simulink model "StSys_StrtCtl"  (R2016b)
settings: configuration reference "CodeGenConfigSet" (kept outside this file)
values from neighbouring files (symbols this model uses):
  Strt_uThresIniMinStrt_C = Calibration.Parameter    [init_StSys_StrtCtl.m]    (also in init_StSys_StrtCtl_SIL.m = Simulink.Parameter)
  StSys_nBlnd_C = Calibration.Parameter    [init_StSys_StrtCtl.m]    (also in init_StSys_StrtCtl_SIL.m = Simulink.Parameter)
  StSys_nThres_C = Calibration.Parameter    [init_StSys_StrtCtl.m]    (also in init_StSys_StrtCtl_SIL.m = Simulink.Parameter)
  StSys_nThresCalc_CUR = Calibration.Parameter    [init_StSys_StrtCtl.m]    (also in init_StSys_StrtCtl_SIL.m = Simulink.Parameter)
  StSys_nThresCalc_CURX = Calibration.Parameter    [init_StSys_StrtCtl.m]    (also in init_StSys_StrtCtl_SIL.m = Simulink.Parameter)
  StSys_stCondActv_C = Calibration.Parameter    [init_StSys_StrtCtl.m]    (also in init_StSys_StrtCtl_SIL.m = Simulink.Parameter)
  StSys_stCondDeactv_C = Calibration.Parameter    [init_StSys_StrtCtl.m]    (also in init_StSys_StrtCtl_SIL.m = Simulink.Parameter)
  StSys_stLogicT50CAN_C = Calibration.Parameter    [init_StSys_StrtCtl.m]    (also in init_StSys_StrtCtl_SIL.m = Simulink.Parameter)
  StSys_stLogicT50EMGCY_C = Calibration.Parameter    [init_StSys_StrtCtl.m]    (also in init_StSys_StrtCtl_SIL.m = Simulink.Parameter)
  StSys_stLogicT50NRM_C = Calibration.Parameter    [init_StSys_StrtCtl.m]    (also in init_StSys_StrtCtl_SIL.m = Simulink.Parameter)
  StSys_stSelectT50CAN_C = Calibration.Parameter    [init_StSys_StrtCtl.m]    (also in init_StSys_StrtCtl_SIL.m = Simulink.Parameter)
  StSys_stSelectT50EMGCY_C = Calibration.Parameter    [init_StSys_StrtCtl.m]    (also in init_StSys_StrtCtl_SIL.m = Simulink.Parameter)
  StSys_stSelectT50NRM_C = Calibration.Parameter    [init_StSys_StrtCtl.m]    (also in init_StSys_StrtCtl_SIL.m = Simulink.Parameter)
  StSys_tiBlnd_C = Calibration.Parameter    [init_StSys_StrtCtl.m]    (also in init_StSys_StrtCtl_SIL.m = Simulink.Parameter)
  StSys_tiStrtON_C = Calibration.Parameter    [init_StSys_StrtCtl.m]    (also in init_StSys_StrtCtl_SIL.m = Simulink.Parameter)
  StSys_vEngCompStrt_C = Calibration.Parameter    [init_StSys_StrtCtl.m]    (also in init_StSys_StrtCtl_SIL.m = Simulink.Parameter)
  StSys_vThresT50CAN_C = Calibration.Parameter    [init_StSys_StrtCtl.m]    (also in init_StSys_StrtCtl_SIL.m = Simulink.Parameter)
  StSys_vThresT50EMGCY_C = Calibration.Parameter    [init_StSys_StrtCtl.m]    (also in init_StSys_StrtCtl_SIL.m = Simulink.Parameter)
  StSys_vThresT50NRM_C = Calibration.Parameter    [init_StSys_StrtCtl.m]    (also in init_StSys_StrtCtl_SIL.m = Simulink.Parameter)
undefined symbols (not defined in the file or in its folder): AirHtState_conv, StSys_StrtCtl_DT, StSys_StrtState_conv
libraries: simulink x201, CXLib x7
(part 2 of 2)

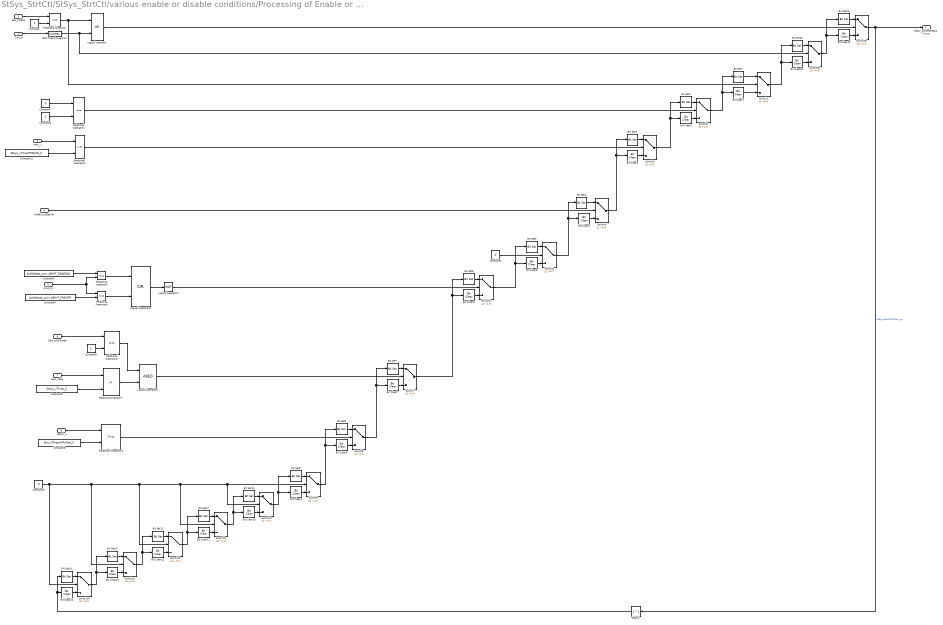
== system StSys_StrtCtl/StSys_StrtCtl/various enable or disable conditions/Processing of Enable or disable conditions for T50CAN ==
  Gbx_stNPos : Inport
  Clth_st : Inport  Port=2
  VehV_v : Inport  Port=3
  HndBrk_stDebVal : Inport  Port=4
  AirHt_st : Inport  Port=5
  Epm_stOpMode : Inport  Port=6
  Epm_nEng : Inport  Port=7
  BattU_u : Inport  Port=8
  Bit Clear1 : simulink/Logic and Bit Operations/Bit Clear  iBit=2
  Bit Clear10 : simulink/Logic and Bit Operations/Bit Clear  iBit=11
  Bit Clear11 : simulink/Logic and Bit Operations/Bit Clear  iBit=12
  Bit Clear12 : simulink/Logic and Bit Operations/Bit Clear  iBit=13
  Bit Clear13 : simulink/Logic and Bit Operations/Bit Clear  iBit=14
  Bit Clear14 : simulink/Logic and Bit Operations/Bit Clear  iBit=15
  Bit Clear2 : simulink/Logic and Bit Operations/Bit Clear  iBit=3
  Bit Clear3 : simulink/Logic and Bit Operations/Bit Clear  iBit=4
  Bit Clear4 : simulink/Logic and Bit Operations/Bit Clear  iBit=5
  Bit Clear41 : simulink/Logic and Bit Operations/Bit Clear  iBit=0
  Bit Clear5 : simulink/Logic and Bit Operations/Bit Clear  iBit=6
  Bit Clear54 : simulink/Logic and Bit Operations/Bit Clear  iBit=1
  Bit Clear6 : simulink/Logic and Bit Operations/Bit Clear  iBit=7
  Bit Clear7 : simulink/Logic and Bit Operations/Bit Clear  iBit=8
  Bit Clear8 : simulink/Logic and Bit Operations/Bit Clear  iBit=9
  Bit Clear9 : simulink/Logic and Bit Operations/Bit Clear  iBit=10
  Bit Set1 : simulink/Logic and Bit Operations/Bit Set  iBit=2
  Bit Set10 : simulink/Logic and Bit Operations/Bit Set  iBit=11
  Bit Set11 : simulink/Logic and Bit Operations/Bit Set  iBit=12
  Bit Set12 : simulink/Logic and Bit Operations/Bit Set  iBit=13
  Bit Set13 : simulink/Logic and Bit Operations/Bit Set  iBit=14
  Bit Set14 : simulink/Logic and Bit Operations/Bit Set  iBit=15
  Bit Set18 : simulink/Logic and Bit Operations/Bit Set  iBit=1
  Bit Set2 : simulink/Logic and Bit Operations/Bit Set  iBit=3
  Bit Set24 : simulink/Logic and Bit Operations/Bit Set  iBit=0
  Bit Set3 : simulink/Logic and Bit Operations/Bit Set  iBit=4
  Bit Set4 : simulink/Logic and Bit Operations/Bit Set  iBit=5
  Bit Set5 : simulink/Logic and Bit Operations/Bit Set  iBit=6
  Bit Set6 : simulink/Logic and Bit Operations/Bit Set  iBit=7
  Bit Set7 : simulink/Logic and Bit Operations/Bit Set  iBit=8
  Bit Set8 : simulink/Logic and Bit Operations/Bit Set  iBit=9
  Bit Set9 : simulink/Logic and Bit Operations/Bit Set  iBit=10
  Constant : Constant  OutDataTypeStr=uint8
  Constant1 : Constant  OutDataTypeStr=uint8
  Constant11 : Constant  Value=StSys_vThresT50CAN_C
  Constant2 : Constant  Value=0  OutDataTypeStr=boolean
  Constant3 : Constant  Value=AirHtState_conv.AIRHT_READING
  Constant4 : Constant  Value=AirHtState_conv.AIRHT_PREHTR
  Constant5 : Constant  OutDataTypeStr=Inherit: Inherit via back propagation
  Constant6 : Constant  Value=0  OutDataTypeStr=boolean
  Constant7 : Constant  Value=0  OutDataTypeStr=uint8
  Constant8 : Constant  Value=Strt_uThresIniMinStrt_C
  Constant9 : Constant  Value=StSys_nThres_C
  Data Type Conversion : DataTypeConversion  OutDataTypeStr=boolean
  Delay2 : Delay  DelayLength=1  InitialCondition=0
  Logical Operator : Logic  Operator=OR  AllPortsSameDT=off  OutDataTypeStr=boolean
  Logical Operator1 : Logic  Operator=NOT  AllPortsSameDT=off  OutDataTypeStr=boolean
  Logical Operator8 : Logic  Operator=OR  AllPortsSameDT=off  OutDataTypeStr=boolean
  Logical Operator9 : Logic  AllPortsSameDT=off  OutDataTypeStr=boolean
  Relational Operator : RelationalOperator  Operator===  OutDataTypeStr=boolean  RndMeth=Simplest  InputSameDT=on
  Relational Operator1 : RelationalOperator  Operator===  OutDataTypeStr=boolean  RndMeth=Simplest  InputSameDT=on
  Relational Operator2 : RelationalOperator  Operator=<=  OutDataTypeStr=boolean  RndMeth=Simplest
  Relational Operator3 : RelationalOperator  OutDataTypeStr=boolean  RndMeth=Simplest
  Relational Operator5 : RelationalOperator  Operator===  OutDataTypeStr=boolean  RndMeth=Simplest
  Relational Operator6 : RelationalOperator  Operator===  OutDataTypeStr=boolean  RndMeth=Simplest
  Relational Operator7 : RelationalOperator  Operator=<  OutDataTypeStr=boolean  RndMeth=Simplest
  Relational Operator8 : RelationalOperator  Operator===  OutDataTypeStr=boolean  RndMeth=Simplest
  Switch{1..14,29,36} (16 alike) : Switch  Criteria=u2 ~= 0  InputSameDT=on
  StSys_stCondT50CAN_mp : Outport
  wires:
  Switch29/1 -> StSys_stCondT50CAN_mp/1, Delay2/1  "StSys_stCondT50CAN_mp"
  Bit Set24/1 -> Switch29/1
  Bit Clear41/1 -> Switch29/3
  Delay2/1 -> Bit Clear14/1, Bit Set14/1
  Switch36/1 -> Bit Clear41/1, Bit Set24/1
  Bit Set18/1 -> Switch36/1
  Bit Clear54/1 -> Switch36/3
  Switch1/1 -> Bit Set18/1, Bit Clear54/1
  Bit Set1/1 -> Switch1/1
  Bit Clear1/1 -> Switch1/3
  Switch2/1 -> Bit Set1/1, Bit Clear1/1
  Bit Set2/1 -> Switch2/1
  Bit Clear2/1 -> Switch2/3
  Switch3/1 -> Bit Clear2/1, Bit Set2/1
  Bit Set3/1 -> Switch3/1
  Bit Clear3/1 -> Switch3/3
  Switch4/1 -> Bit Set3/1, Bit Clear3/1
  Bit Set4/1 -> Switch4/1
  Bit Clear4/1 -> Switch4/3
  Switch5/1 -> Bit Set4/1, Bit Clear4/1
  Bit Set5/1 -> Switch5/1
  Bit Clear5/1 -> Switch5/3
  Switch6/1 -> Bit Set5/1, Bit Clear5/1
  Bit Set6/1 -> Switch6/1
  Bit Clear6/1 -> Switch6/3
  Switch7/1 -> Bit Set6/1, Bit Clear6/1
  Bit Set7/1 -> Switch7/1
  Bit Clear7/1 -> Switch7/3
  Switch8/1 -> Bit Set7/1, Bit Clear7/1
  Bit Set8/1 -> Switch8/1
  Bit Clear8/1 -> Switch8/3
  Switch9/1 -> Bit Set8/1, Bit Clear8/1
  Bit Set9/1 -> Switch9/1
  Bit Clear9/1 -> Switch9/3
  Switch10/1 -> Bit Set9/1, Bit Clear9/1
  Bit Set10/1 -> Switch10/1
  Bit Clear10/1 -> Switch10/3
  Switch11/1 -> Bit Clear10/1, Bit Set10/1
  Bit Set11/1 -> Switch11/1
  Bit Clear11/1 -> Switch11/3
  Switch12/1 -> Bit Set11/1, Bit Clear11/1
  Bit Set12/1 -> Switch12/1
  Bit Clear12/1 -> Switch12/3
  Switch13/1 -> Bit Set12/1, Bit Clear12/1
  Bit Set13/1 -> Switch13/1
  Bit Clear13/1 -> Switch13/3
  Switch14/1 -> Bit Set13/1, Bit Clear13/1
  Bit Set14/1 -> Switch14/1
  Bit Clear14/1 -> Switch14/3
  Gbx_stNPos/1 -> Relational Operator/1
  Constant/1 -> Relational Operator/2
  Logical Operator/1 -> Switch29/2
  Clth_st/1 -> Data Type Conversion/1
  Relational Operator/1 -> Switch1/2, Logical Operator/1
  Constant7/1 -> Relational Operator1/1
  Constant1/1 -> Relational Operator1/2
  Relational Operator1/1 -> Switch2/2
  VehV_v/1 -> Relational Operator2/1
  Constant11/1 -> Relational Operator2/2
  Relational Operator2/1 -> Switch3/2
  HndBrk_stDebVal/1 -> Switch4/2
  Constant2/1 -> Switch5/2
  AirHt_st/1 -> Relational Operator5/2, Relational Operator6/1
  Constant3/1 -> Relational Operator5/1
  Constant4/1 -> Relational Operator6/2
  Relational Operator5/1 -> Logical Operator8/1
  Relational Operator6/1 -> Logical Operator8/2
  Logical Operator8/1 -> Logical Operator1/1
  Epm_nEng/1 -> Relational Operator7/1
  Constant9/1 -> Relational Operator7/2
  Relational Operator7/1 -> Logical Operator9/2
  Epm_stOpMode/1 -> Relational Operator8/1
  Constant5/1 -> Relational Operator8/2
  Relational Operator8/1 -> Logical Operator9/1
  Logical Operator9/1 -> Switch7/2
  Constant6/1 -> Switch14/2, Switch13/2, Switch12/2, Switch11/2, Switch10/2, Switch9/2
  Logical Operator1/1 -> Switch6/2
  Data Type Conversion/1 -> Switch36/2, Logical Operator/2
  BattU_u/1 -> Relational Operator3/1
  Constant8/1 -> Relational Operator3/2
  Relational Operator3/1 -> Switch8/2

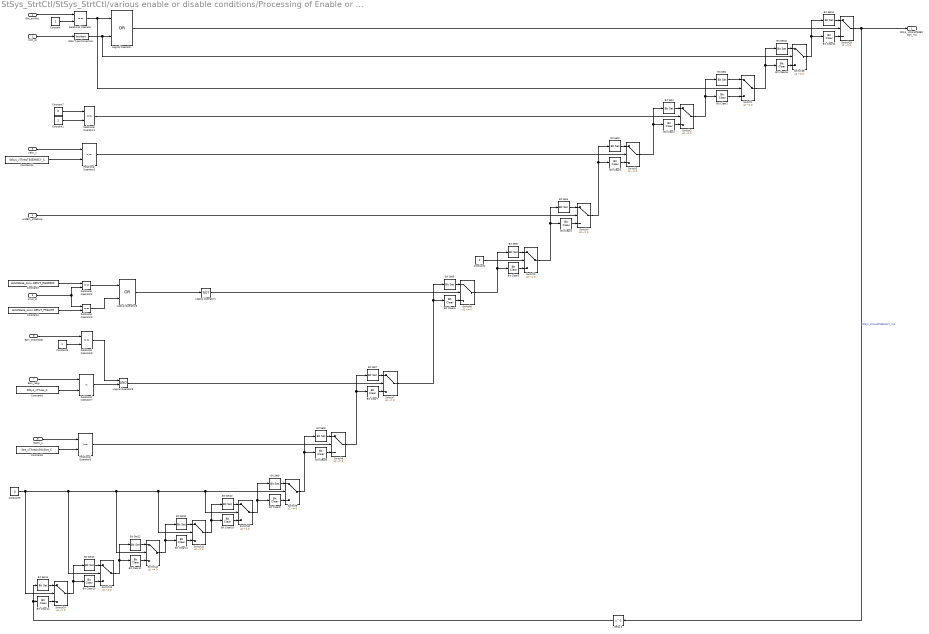
== system StSys_StrtCtl/StSys_StrtCtl/various enable or disable conditions/Processing of Enable or disable conditions for T50EMGCY ==
  Gbx_stNPos : Inport
  Clth_st : Inport  Port=2
  VehV_v : Inport  Port=3
  HndBrk_stDebVal : Inport  Port=4
  AirHt_st : Inport  Port=5
  Epm_stOpMode : Inport  Port=6
  Epm_nEng : Inport  Port=7
  BattU_u : Inport  Port=8
  Bit Clear1 : simulink/Logic and Bit Operations/Bit Clear  iBit=2
  Bit Clear10 : simulink/Logic and Bit Operations/Bit Clear  iBit=11
  Bit Clear11 : simulink/Logic and Bit Operations/Bit Clear  iBit=12
  Bit Clear12 : simulink/Logic and Bit Operations/Bit Clear  iBit=13
  Bit Clear13 : simulink/Logic and Bit Operations/Bit Clear  iBit=14
  Bit Clear14 : simulink/Logic and Bit Operations/Bit Clear  iBit=15
  Bit Clear2 : simulink/Logic and Bit Operations/Bit Clear  iBit=3
  Bit Clear3 : simulink/Logic and Bit Operations/Bit Clear  iBit=4
  Bit Clear4 : simulink/Logic and Bit Operations/Bit Clear  iBit=5
  Bit Clear41 : simulink/Logic and Bit Operations/Bit Clear  iBit=0
  Bit Clear5 : simulink/Logic and Bit Operations/Bit Clear  iBit=6
  Bit Clear54 : simulink/Logic and Bit Operations/Bit Clear  iBit=1
  Bit Clear6 : simulink/Logic and Bit Operations/Bit Clear  iBit=7
  Bit Clear7 : simulink/Logic and Bit Operations/Bit Clear  iBit=8
  Bit Clear8 : simulink/Logic and Bit Operations/Bit Clear  iBit=9
  Bit Clear9 : simulink/Logic and Bit Operations/Bit Clear  iBit=10
  Bit Set1 : simulink/Logic and Bit Operations/Bit Set  iBit=2
  Bit Set10 : simulink/Logic and Bit Operations/Bit Set  iBit=11
  Bit Set11 : simulink/Logic and Bit Operations/Bit Set  iBit=12
  Bit Set12 : simulink/Logic and Bit Operations/Bit Set  iBit=13
  Bit Set13 : simulink/Logic and Bit Operations/Bit Set  iBit=14
  Bit Set14 : simulink/Logic and Bit Operations/Bit Set  iBit=15
  Bit Set18 : simulink/Logic and Bit Operations/Bit Set  iBit=1
  Bit Set2 : simulink/Logic and Bit Operations/Bit Set  iBit=3
  Bit Set24 : simulink/Logic and Bit Operations/Bit Set  iBit=0
  Bit Set3 : simulink/Logic and Bit Operations/Bit Set  iBit=4
  Bit Set4 : simulink/Logic and Bit Operations/Bit Set  iBit=5
  Bit Set5 : simulink/Logic and Bit Operations/Bit Set  iBit=6
  Bit Set6 : simulink/Logic and Bit Operations/Bit Set  iBit=7
  Bit Set7 : simulink/Logic and Bit Operations/Bit Set  iBit=8
  Bit Set8 : simulink/Logic and Bit Operations/Bit Set  iBit=9
  Bit Set9 : simulink/Logic and Bit Operations/Bit Set  iBit=10
  Constant : Constant  OutDataTypeStr=uint8
  Constant1 : Constant  OutDataTypeStr=uint8
  Constant11 : Constant  Value=StSys_vThresT50EMGCY_C
  Constant2 : Constant  Value=0  OutDataTypeStr=boolean
  Constant3 : Constant  Value=AirHtState_conv.AIRHT_READING
  Constant4 : Constant  Value=AirHtState_conv.AIRHT_PREHTR
  Constant5 : Constant  OutDataTypeStr=Inherit: Inherit via back propagation
  Constant6 : Constant  Value=0  OutDataTypeStr=boolean
  Constant7 : Constant  Value=0  OutDataTypeStr=uint8
  Constant8 : Constant  Value=Strt_uThresIniMinStrt_C
  Constant9 : Constant  Value=StSys_nThres_C
  Data Type Conversion : DataTypeConversion  OutDataTypeStr=boolean
  Delay2 : Delay  DelayLength=1  InitialCondition=0
  Logical Operator : Logic  Operator=OR  AllPortsSameDT=off  OutDataTypeStr=boolean
  Logical Operator1 : Logic  Operator=NOT  AllPortsSameDT=off  OutDataTypeStr=boolean
  Logical Operator8 : Logic  Operator=OR  AllPortsSameDT=off  OutDataTypeStr=boolean
  Logical Operator9 : Logic  AllPortsSameDT=off  OutDataTypeStr=boolean
  Relational Operator : RelationalOperator  Operator===  OutDataTypeStr=boolean  RndMeth=Simplest  InputSameDT=on
  Relational Operator1 : RelationalOperator  Operator===  OutDataTypeStr=boolean  RndMeth=Simplest  InputSameDT=on
  Relational Operator2 : RelationalOperator  Operator=<=  OutDataTypeStr=boolean  RndMeth=Simplest
  Relational Operator3 : RelationalOperator  OutDataTypeStr=boolean  RndMeth=Simplest
  Relational Operator5 : RelationalOperator  Operator===  OutDataTypeStr=boolean  RndMeth=Simplest
  Relational Operator6 : RelationalOperator  Operator===  OutDataTypeStr=boolean  RndMeth=Simplest
  Relational Operator7 : RelationalOperator  Operator=<  OutDataTypeStr=boolean  RndMeth=Simplest
  Relational Operator8 : RelationalOperator  Operator===  OutDataTypeStr=boolean  RndMeth=Simplest  InputSameDT=on
  Switch{1..14,29,36} (16 alike) : Switch  Criteria=u2 ~= 0  InputSameDT=on
  StSys_stCondT50EMGCY_mp : Outport
  wires:
  Switch29/1 -> StSys_stCondT50EMGCY_mp/1, Delay2/1  "StSys_stCondT50EMGCY_mp"
  Bit Set24/1 -> Switch29/1
  Bit Clear41/1 -> Switch29/3
  Delay2/1 -> Bit Clear14/1, Bit Set14/1
  Switch36/1 -> Bit Clear41/1, Bit Set24/1
  Bit Set18/1 -> Switch36/1
  Bit Clear54/1 -> Switch36/3
  Switch1/1 -> Bit Set18/1, Bit Clear54/1
  Bit Set1/1 -> Switch1/1
  Bit Clear1/1 -> Switch1/3
  Switch2/1 -> Bit Set1/1, Bit Clear1/1
  Bit Set2/1 -> Switch2/1
  Bit Clear2/1 -> Switch2/3
  Switch3/1 -> Bit Clear2/1, Bit Set2/1
  Bit Set3/1 -> Switch3/1
  Bit Clear3/1 -> Switch3/3
  Switch4/1 -> Bit Set3/1, Bit Clear3/1
  Bit Set4/1 -> Switch4/1
  Bit Clear4/1 -> Switch4/3
  Switch5/1 -> Bit Set4/1, Bit Clear4/1
  Bit Set5/1 -> Switch5/1
  Bit Clear5/1 -> Switch5/3
  Switch6/1 -> Bit Set5/1, Bit Clear5/1
  Bit Set6/1 -> Switch6/1
  Bit Clear6/1 -> Switch6/3
  Switch7/1 -> Bit Set6/1, Bit Clear6/1
  Bit Set7/1 -> Switch7/1
  Bit Clear7/1 -> Switch7/3
  Switch8/1 -> Bit Set7/1, Bit Clear7/1
  Bit Set8/1 -> Switch8/1
  Bit Clear8/1 -> Switch8/3
  Switch9/1 -> Bit Set8/1, Bit Clear8/1
  Bit Set9/1 -> Switch9/1
  Bit Clear9/1 -> Switch9/3
  Switch10/1 -> Bit Set9/1, Bit Clear9/1
  Bit Set10/1 -> Switch10/1
  Bit Clear10/1 -> Switch10/3
  Switch11/1 -> Bit Clear10/1, Bit Set10/1
  Bit Set11/1 -> Switch11/1
  Bit Clear11/1 -> Switch11/3
  Switch12/1 -> Bit Set11/1, Bit Clear11/1
  Bit Set12/1 -> Switch12/1
  Bit Clear12/1 -> Switch12/3
  Switch13/1 -> Bit Set12/1, Bit Clear12/1
  Bit Set13/1 -> Switch13/1
  Bit Clear13/1 -> Switch13/3
  Switch14/1 -> Bit Set13/1, Bit Clear13/1
  Bit Set14/1 -> Switch14/1
  Bit Clear14/1 -> Switch14/3
  Gbx_stNPos/1 -> Relational Operator/1
  Constant/1 -> Relational Operator/2
  Logical Operator/1 -> Switch29/2
  Clth_st/1 -> Data Type Conversion/1
  Relational Operator/1 -> Switch1/2, Logical Operator/1
  Constant7/1 -> Relational Operator1/1
  Constant1/1 -> Relational Operator1/2
  Relational Operator1/1 -> Switch2/2
  VehV_v/1 -> Relational Operator2/1
  Constant11/1 -> Relational Operator2/2
  Relational Operator2/1 -> Switch3/2
  HndBrk_stDebVal/1 -> Switch4/2
  Constant2/1 -> Switch5/2
  AirHt_st/1 -> Relational Operator6/1, Relational Operator5/2
  Constant3/1 -> Relational Operator5/1
  Constant4/1 -> Relational Operator6/2
  Relational Operator5/1 -> Logical Operator8/1
  Relational Operator6/1 -> Logical Operator8/2
  Logical Operator8/1 -> Logical Operator1/1
  Epm_nEng/1 -> Relational Operator7/1
  Constant9/1 -> Relational Operator7/2
  Relational Operator7/1 -> Logical Operator9/2
  Epm_stOpMode/1 -> Relational Operator8/1
  Constant5/1 -> Relational Operator8/2
  Relational Operator8/1 -> Logical Operator9/1
  Logical Operator9/1 -> Switch7/2
  Constant6/1 -> Switch14/2, Switch13/2, Switch12/2, Switch11/2, Switch10/2, Switch9/2
  Logical Operator1/1 -> Switch6/2
  Data Type Conversion/1 -> Switch36/2, Logical Operator/2
  BattU_u/1 -> Relational Operator3/1
  Constant8/1 -> Relational Operator3/2
  Relational Operator3/1 -> Switch8/2

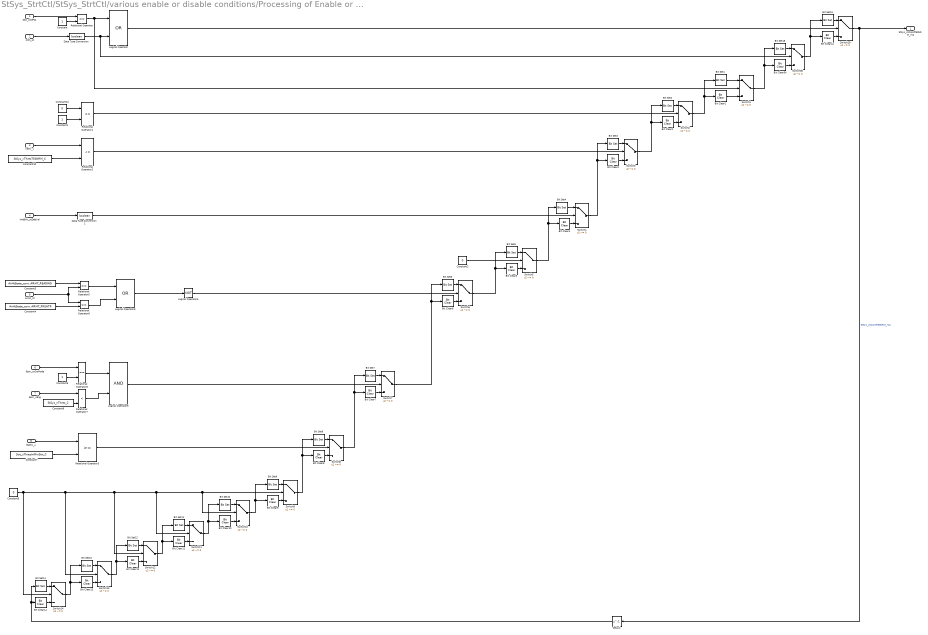
== system StSys_StrtCtl/StSys_StrtCtl/various enable or disable conditions/Processing of Enable or disable conditions for T50NRM ==
  Gbx_stNPos : Inport
  Clth_st : Inport  Port=2
  VehV_v : Inport  Port=3
  HndBrk_stDebVal : Inport  Port=4
  AirHt_st : Inport  Port=5
  Epm_stOpMode : Inport  Port=6
  Epm_nEng : Inport  Port=7
  BattU_u : Inport  Port=8
  Bit Clear1 : simulink/Logic and Bit Operations/Bit Clear  iBit=2
  Bit Clear10 : simulink/Logic and Bit Operations/Bit Clear  iBit=11
  Bit Clear11 : simulink/Logic and Bit Operations/Bit Clear  iBit=12
  Bit Clear12 : simulink/Logic and Bit Operations/Bit Clear  iBit=13
  Bit Clear13 : simulink/Logic and Bit Operations/Bit Clear  iBit=14
  Bit Clear14 : simulink/Logic and Bit Operations/Bit Clear  iBit=15
  Bit Clear2 : simulink/Logic and Bit Operations/Bit Clear  iBit=3
  Bit Clear3 : simulink/Logic and Bit Operations/Bit Clear  iBit=4
  Bit Clear4 : simulink/Logic and Bit Operations/Bit Clear  iBit=5
  Bit Clear41 : simulink/Logic and Bit Operations/Bit Clear  iBit=0
  Bit Clear5 : simulink/Logic and Bit Operations/Bit Clear  iBit=6
  Bit Clear54 : simulink/Logic and Bit Operations/Bit Clear  iBit=1
  Bit Clear6 : simulink/Logic and Bit Operations/Bit Clear  iBit=7
  Bit Clear7 : simulink/Logic and Bit Operations/Bit Clear  iBit=8
  Bit Clear8 : simulink/Logic and Bit Operations/Bit Clear  iBit=9
  Bit Clear9 : simulink/Logic and Bit Operations/Bit Clear  iBit=10
  Bit Set1 : simulink/Logic and Bit Operations/Bit Set  iBit=2
  Bit Set10 : simulink/Logic and Bit Operations/Bit Set  iBit=11
  Bit Set11 : simulink/Logic and Bit Operations/Bit Set  iBit=12
  Bit Set12 : simulink/Logic and Bit Operations/Bit Set  iBit=13
  Bit Set13 : simulink/Logic and Bit Operations/Bit Set  iBit=14
  Bit Set14 : simulink/Logic and Bit Operations/Bit Set  iBit=15
  Bit Set18 : simulink/Logic and Bit Operations/Bit Set  iBit=1
  Bit Set2 : simulink/Logic and Bit Operations/Bit Set  iBit=3
  Bit Set24 : simulink/Logic and Bit Operations/Bit Set  iBit=0
  Bit Set3 : simulink/Logic and Bit Operations/Bit Set  iBit=4
  Bit Set4 : simulink/Logic and Bit Operations/Bit Set  iBit=5
  Bit Set5 : simulink/Logic and Bit Operations/Bit Set  iBit=6
  Bit Set6 : simulink/Logic and Bit Operations/Bit Set  iBit=7
  Bit Set7 : simulink/Logic and Bit Operations/Bit Set  iBit=8
  Bit Set8 : simulink/Logic and Bit Operations/Bit Set  iBit=9
  Bit Set9 : simulink/Logic and Bit Operations/Bit Set  iBit=10
  Constant : Constant  OutDataTypeStr=Inherit: Inherit via back propagation
  Constant1 : Constant  OutDataTypeStr=uint8
  Constant10 : Constant  Value=StSys_vThresT50NRM_C
  Constant12 : Constant  Value=0  OutDataTypeStr=uint8
  Constant2 : Constant  Value=0  OutDataTypeStr=boolean
  Constant3 : Constant  Value=AirHtState_conv.AIRHT_READING
  Constant4 : Constant  Value=AirHtState_conv.AIRHT_PREHTR
  Constant5 : Constant  OutDataTypeStr=Inherit: Inherit via back propagation
  Constant6 : Constant  Value=0  OutDataTypeStr=boolean
  Constant7 : Constant  Value=Strt_uThresIniMinStrt_C
  Constant9 : Constant  Value=StSys_nThres_C
  Data Type Conversion : DataTypeConversion  OutDataTypeStr=boolean
  Data Type Conversion1 : DataTypeConversion  OutDataTypeStr=boolean
  Delay2 : Delay  DelayLength=1  InitialCondition=0
  Logical Operator : Logic  Operator=OR  AllPortsSameDT=off  OutDataTypeStr=boolean
  Logical Operator5 : Logic  Operator=NOT  AllPortsSameDT=off  OutDataTypeStr=boolean
  Logical Operator8 : Logic  Operator=OR  AllPortsSameDT=off  OutDataTypeStr=boolean
  Logical Operator9 : Logic  AllPortsSameDT=off  OutDataTypeStr=boolean
  Relational Operator : RelationalOperator  Operator===  OutDataTypeStr=boolean  RndMeth=Simplest  InputSameDT=on
  Relational Operator1 : RelationalOperator  Operator===  OutDataTypeStr=boolean  RndMeth=Simplest  InputSameDT=on
  Relational Operator2 : RelationalOperator  Operator=<=  OutDataTypeStr=boolean  RndMeth=Simplest
  Relational Operator3 : RelationalOperator  OutDataTypeStr=boolean  RndMeth=Simplest
  Relational Operator5 : RelationalOperator  Operator===  OutDataTypeStr=boolean  RndMeth=Simplest
  Relational Operator6 : RelationalOperator  Operator===  OutDataTypeStr=boolean  RndMeth=Simplest
  Relational Operator7 : RelationalOperator  Operator=<  OutDataTypeStr=boolean  RndMeth=Simplest
  Relational Operator8 : RelationalOperator  Operator===  OutDataTypeStr=boolean  RndMeth=Simplest  InputSameDT=on
  Switch{1..14,29,36} (16 alike) : Switch  Criteria=u2 ~= 0  InputSameDT=on
  StSys_stCondT50NRM_mp : Outport
  wires:
  Switch29/1 -> StSys_stCondT50NRM_mp/1, Delay2/1  "StSys_stCondT50NRM_mp"
  Bit Set24/1 -> Switch29/1
  Bit Clear41/1 -> Switch29/3
  Delay2/1 -> Bit Clear14/1, Bit Set14/1
  Switch36/1 -> Bit Clear41/1, Bit Set24/1
  Bit Set18/1 -> Switch36/1
  Bit Clear54/1 -> Switch36/3
  Switch1/1 -> Bit Set18/1, Bit Clear54/1
  Bit Set1/1 -> Switch1/1
  Bit Clear1/1 -> Switch1/3
  Switch2/1 -> Bit Set1/1, Bit Clear1/1
  Bit Set2/1 -> Switch2/1
  Bit Clear2/1 -> Switch2/3
  Switch3/1 -> Bit Clear2/1, Bit Set2/1
  Bit Set3/1 -> Switch3/1
  Bit Clear3/1 -> Switch3/3
  Switch4/1 -> Bit Set3/1, Bit Clear3/1
  Bit Set4/1 -> Switch4/1
  Bit Clear4/1 -> Switch4/3
  Switch5/1 -> Bit Set4/1, Bit Clear4/1
  Bit Set5/1 -> Switch5/1
  Bit Clear5/1 -> Switch5/3
  Switch6/1 -> Bit Set5/1, Bit Clear5/1
  Bit Set6/1 -> Switch6/1
  Bit Clear6/1 -> Switch6/3
  Switch7/1 -> Bit Set6/1, Bit Clear6/1
  Bit Set7/1 -> Switch7/1
  Bit Clear7/1 -> Switch7/3
  Switch8/1 -> Bit Set7/1, Bit Clear7/1
  Bit Set8/1 -> Switch8/1
  Bit Clear8/1 -> Switch8/3
  Switch9/1 -> Bit Set8/1, Bit Clear8/1
  Bit Set9/1 -> Switch9/1
  Bit Clear9/1 -> Switch9/3
  Switch10/1 -> Bit Set9/1, Bit Clear9/1
  Bit Set10/1 -> Switch10/1
  Bit Clear10/1 -> Switch10/3
  Switch11/1 -> Bit Clear10/1, Bit Set10/1
  Bit Set11/1 -> Switch11/1
  Bit Clear11/1 -> Switch11/3
  Switch12/1 -> Bit Set11/1, Bit Clear11/1
  Bit Set12/1 -> Switch12/1
  Bit Clear12/1 -> Switch12/3
  Switch13/1 -> Bit Set12/1, Bit Clear12/1
  Bit Set13/1 -> Switch13/1
  Bit Clear13/1 -> Switch13/3
  Switch14/1 -> Bit Set13/1, Bit Clear13/1
  Bit Set14/1 -> Switch14/1
  Bit Clear14/1 -> Switch14/3
  Gbx_stNPos/1 -> Relational Operator/1
  Constant/1 -> Relational Operator/2
  Logical Operator/1 -> Switch29/2
  Clth_st/1 -> Data Type Conversion/1
  Relational Operator/1 -> Switch1/2, Logical Operator/1
  Constant12/1 -> Relational Operator1/1
  Constant1/1 -> Relational Operator1/2
  Relational Operator1/1 -> Switch2/2
  VehV_v/1 -> Relational Operator2/1
  Constant10/1 -> Relational Operator2/2
  Relational Operator2/1 -> Switch3/2
  HndBrk_stDebVal/1 -> Data Type Conversion1/1
  Constant2/1 -> Switch5/2
  AirHt_st/1 -> Relational Operator5/2, Relational Operator6/1
  Constant3/1 -> Relational Operator5/1
  Constant4/1 -> Relational Operator6/2
  Relational Operator5/1 -> Logical Operator8/1
  Relational Operator6/1 -> Logical Operator8/2
  Logical Operator8/1 -> Logical Operator5/1
  Epm_nEng/1 -> Relational Operator7/1
  Constant9/1 -> Relational Operator7/2
  Relational Operator7/1 -> Logical Operator9/2
  Epm_stOpMode/1 -> Relational Operator8/1
  Constant5/1 -> Relational Operator8/2
  Relational Operator8/1 -> Logical Operator9/1
  Logical Operator9/1 -> Switch7/2
  Constant6/1 -> Switch9/2, Switch10/2, Switch11/2, Switch12/2, Switch13/2, Switch14/2
  Logical Operator5/1 -> Switch6/2
  Data Type Conversion/1 -> Switch36/2, Logical Operator/2
  Data Type Conversion1/1 -> Switch4/2
  BattU_u/1 -> Relational Operator3/1
  Constant7/1 -> Relational Operator3/2
  Relational Operator3/1 -> Switch8/2
